simulink model "Problem9"  (R2020b)
settings: Solver=VariableStepAuto  StartTime=0.0  StopTime=10.0  RelTol=1e-3
values from neighbouring files (symbols this model uses):
  b = 0.1    [Problem9_Startup.m]
  J = 0.01    [Problem9_Startup.m]
  K = 0.01    [Problem9_Startup.m]
  L = 0.5    [Problem9_Startup.m]
  R = 1    [Problem9_Startup.m]
settings Model: Creator=Shirish  LastModifiedBy=Shirish

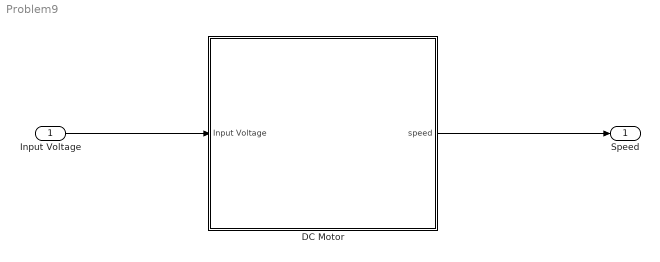
== system Problem9 ==
  Input Voltage : Inport
  DC Motor : Subsystem
  Speed : Outport
  wires:
  Input Voltage/1 -> DC Motor/1(Input Voltage)
  DC Motor/1(speed) -> Speed/1

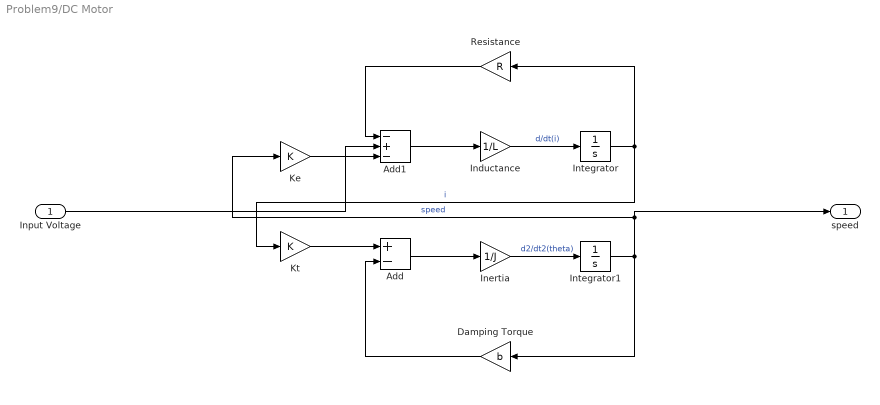
== system Problem9/DC Motor ==
  Input Voltage : Inport
  Add : Sum  Inputs=+-
  Add1 : Sum  Inputs=-+-
  Damping Torque : Gain  Gain=b
  Inductance : Gain  Gain=1/L
  Inertia : Gain  Gain=1/J
  Integrator : Integrator
  Integrator1 : Integrator
  Ke : Gain  Gain=K
  Kt : Gain  Gain=K
  Resistance : Gain  Gain=R
  speed : Outport
  wires:
  Inertia/1 -> Integrator1/1  "d2/dt2(theta)"
  Kt/1 -> Add/1
  Ke/1 -> Add1/3
  Inductance/1 -> Integrator/1  "d/dt(i)"
  Integrator1/1 -> speed/1, Ke/1, Damping Torque/1  "speed"
  Damping Torque/1 -> Add/2
  Resistance/1 -> Add1/1
  Integrator/1 -> Kt/1, Resistance/1  "i"
  Add1/1 -> Inductance/1
  Add/1 -> Inertia/1
  Input Voltage/1 -> Add1/2
